simulink model "Cowley436PDController"  (R2022b)
settings: Solver=VariableStepAuto  StartTime=0.0  StopTime=10.0  RelTol=1e-3
undefined symbols (not defined in the file or in its folder): kd, kp
libraries: simulink x3
settings Model: Creator=mattcowley  LastModifiedBy=mattcowley

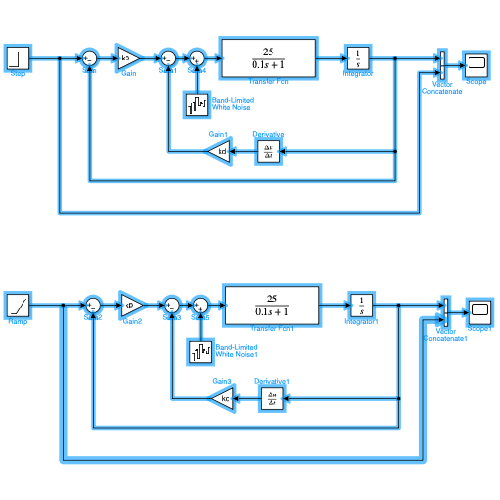
[thumbnail: Simulink's stored preview of the top-level diagram]
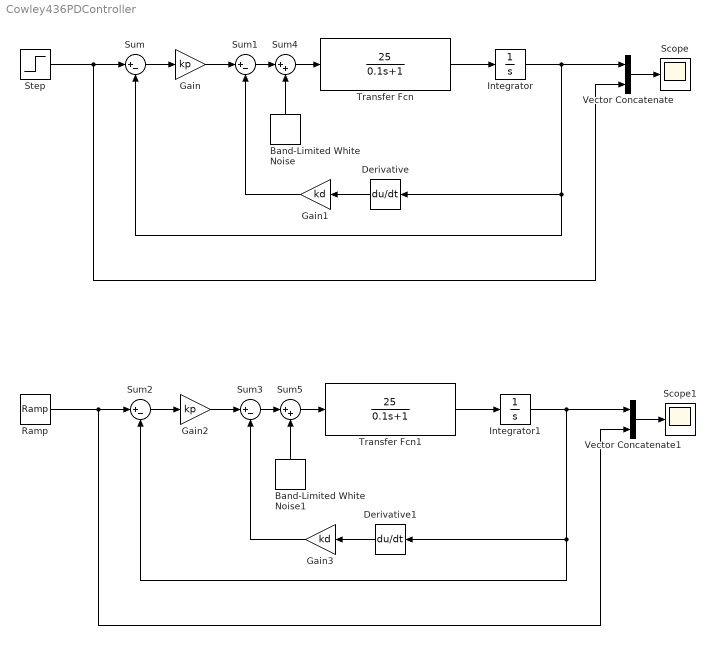
== system Cowley436PDController ==
  Band-Limited White Noise : simulink/Sources/Band-Limited White Noise  Cov=.001  Ts=0.1  seed=[23341]
  Band-Limited White Noise1 : simulink/Sources/Band-Limited White Noise  Cov=.001  Ts=0.1  seed=[23341]
  Derivative : Derivative
  Derivative1 : Derivative
  Gain : Gain  Gain=kp
  Gain1 : Gain  Gain=kd
  Gain2 : Gain  Gain=kp
  Gain3 : Gain  Gain=kd
  Integrator : Integrator
  Integrator1 : Integrator
  Ramp : simulink/Sources/Ramp  slope=pi  start=0  InitialOutput=0
  Scope : Scope
  Scope1 : Scope
  Step : Step  After=pi  SampleTime=0
  Sum{,1..3} (4 alike) : Sum  Inputs=|+-
  Sum4 : Sum  Inputs=|++
  Sum5 : Sum  Inputs=|++
  Transfer Fcn : TransferFcn  Numerator=25  Denominator=[0.1 1]
  Transfer Fcn1 : TransferFcn  Numerator=25  Denominator=[0.1 1]
  Vector Concatenate : Concatenate
  Vector Concatenate1 : Concatenate
  wires:
  Step/1 -> Vector Concatenate/2, Sum/1
  Sum/1 -> Gain/1
  Gain/1 -> Sum1/1
  Derivative/1 -> Gain1/1
  Gain1/1 -> Sum1/2
  Integrator/1 -> Sum/2, Derivative/1, Vector Concatenate/1
  Vector Concatenate/1 -> Scope/1
  Transfer Fcn/1 -> Integrator/1
  Gain2/1 -> Sum3/1
  Sum2/1 -> Gain2/1
  Gain3/1 -> Sum3/2
  Vector Concatenate1/1 -> Scope1/1
  Integrator1/1 -> Sum2/2, Derivative1/1, Vector Concatenate1/1
  Derivative1/1 -> Gain3/1
  Ramp/1 -> Vector Concatenate1/2, Sum2/1
  Transfer Fcn1/1 -> Integrator1/1
  Sum1/1 -> Sum4/1
  Sum4/1 -> Transfer Fcn/1
  Band-Limited White Noise/1 -> Sum4/2
  Band-Limited White Noise1/1 -> Sum5/2
  Sum3/1 -> Sum5/1
  Sum5/1 -> Transfer Fcn1/1
